simulink model "sum3"  (R2020b)
settings: Solver=VariableStepAuto  StartTime=0.0  StopTime=10.0  RelTol=1e-3
undefined symbols (not defined in the file or in its folder): b, m
settings Model: Creator=Shivani  LastModifiedBy=Shivani

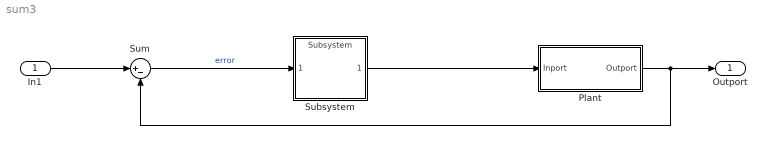
== system sum3 ==
  In1 : Inport
  Plant : Subsystem
  Subsystem : ModelReference  ModelNameDialog=Subsystem  SimulationMode=Normal  ModelReferenceVersion=1.12
  Sum : Sum  Inputs=|+-
  Outport : Outport
  wires:
  Plant/1(Outport) -> Outport/1, Sum/2
  Subsystem/1 -> Plant/1(Inport)
  Sum/1 -> Subsystem/1  "error"
  In1/1 -> Sum/1

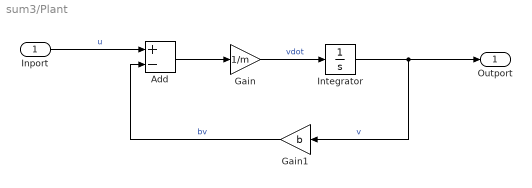
== system sum3/Plant ==
  Inport : Inport
  Add : Sum  Inputs=+-
  Gain : Gain  Gain=1/m
  Gain1 : Gain  Gain=b
  Integrator : Integrator
  Outport : Outport
  wires:
  Gain1/1 -> Add/2  "bv"
  Add/1 -> Gain/1
  Integrator/1 -> Outport/1, Gain1/1  "v"
  Gain/1 -> Integrator/1  "vdot"
  Inport/1 -> Add/1  "u"
